simulink model "21Control_velocidad_PI"  (R2023a)
settings: Solver=VariableStepAuto  StartTime=0.0  StopTime=20  RelTol=1e-3
settings Model: Creator=alexo  LastModifiedBy=alexo

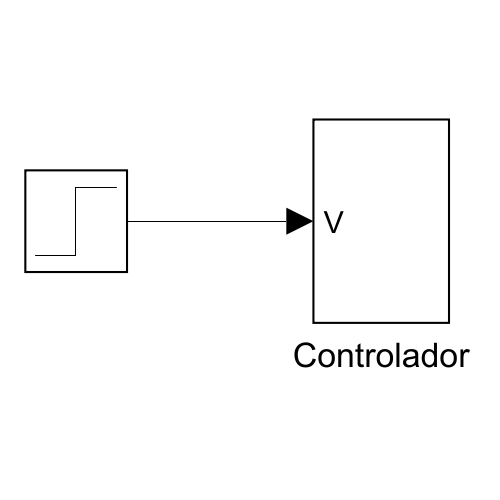
[thumbnail: Simulink's stored preview of the top-level diagram]
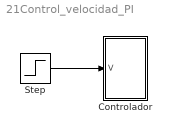
== system 21Control_velocidad_PI ==
  Controlador : Subsystem  mask{Kp=8, Td=3, Ti=0.5}
  Step : Step  Time=2  SampleTime=5
  wires:
  Step/1 -> Controlador/1(V)

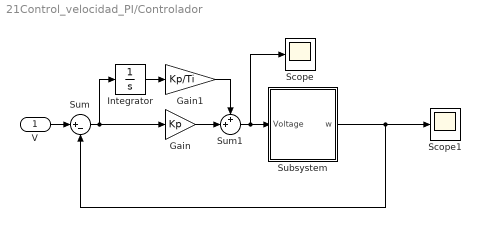
== system 21Control_velocidad_PI/Controlador ==
  V : Inport
  Gain : Gain  Gain=Kp
  Gain1 : Gain  Gain=Kp/Ti
  Integrator : Integrator
  Scope : Scope
  Scope1 : Scope
  Subsystem : Subsystem  mask{J=0.01, b=0.1, Kg=0.01, Km=0.01, R=1, L=0.5}
  Sum : Sum  Inputs=|+-
  Sum1 : Sum  Inputs=++|
  wires:
  Sum/1 -> Integrator/1, Gain/1
  Gain1/1 -> Sum1/1
  Subsystem/1(w) -> Scope1/1, Sum/2
  Sum1/1 -> Scope/1, Subsystem/1(Voltage)
  Integrator/1 -> Gain1/1
  Gain/1 -> Sum1/2
  V/1 -> Sum/1

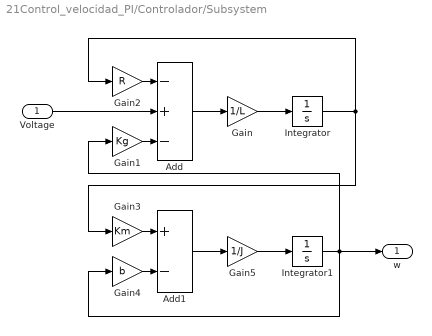
== system 21Control_velocidad_PI/Controlador/Subsystem ==
  Voltage : Inport
  Add : Sum  Inputs=-+-
  Add1 : Sum  Inputs=+-
  Gain : Gain  Gain=1/L
  Gain1 : Gain  Gain=Kg
  Gain2 : Gain  Gain=R
  Gain3 : Gain  Gain=Km
  Gain4 : Gain  Gain=b
  Gain5 : Gain  Gain=1/J
  Integrator : Integrator
  Integrator1 : Integrator
  w : Outport
  wires:
  Gain/1 -> Integrator/1
  Gain2/1 -> Add/1
  Integrator/1 -> Gain3/1, Gain2/1
  Gain4/1 -> Add1/2
  Add/1 -> Gain/1
  Gain1/1 -> Add/3
  Gain5/1 -> Integrator1/1
  Gain3/1 -> Add1/1
  Add1/1 -> Gain5/1
  Integrator1/1 -> w/1, Gain1/1, Gain4/1
  Voltage/1 -> Add/2
